simulink model "CH"  (R2024a)
settings: Solver=VariableStepAuto  StartTime=0.0  StopTime=7000  FixedStep=1e-3  RelTol=1e-3
libraries: visionfilter x1, commrandsrc3 x1
(part 1 of 3)
settings Model: Creator=Eng. Amr  LastModifiedBy=Eng. Amr

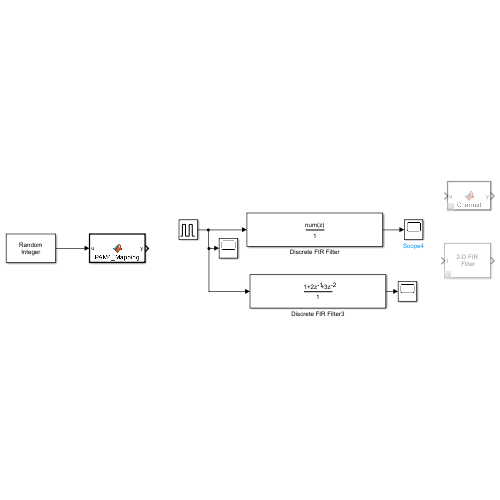
[thumbnail: Simulink's stored preview of the top-level diagram]
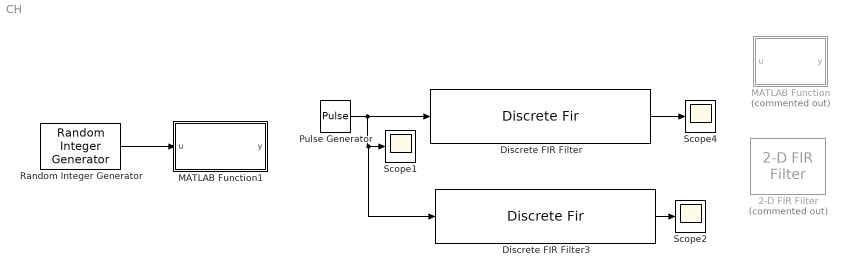
== system CH ==
  2-D FIR Filter : visionfilter/2-D FIR Filter  Commented=on  separable=off  filtSrc=Specify via dialog  filterMtrx=[1 0; 0 -1]  verticalFilter=[4 0]  horizontalFilter=[4 0]  outSize=Full  padType=Constant  padSrc=Specify via dialog  padVal=0  method=Convolution  firstCoeffMode=Specify word length  firstCoeffWordLength=16  firstCoeffFracLength=14  firstCoeffSignedness=Signed  firstCoeffLastDataTypeStr=fixdt(1,16)  outputSignedness=Auto  accumLastDataTypeStr=Inherit: Same as product output  prodOutputMode=Binary point scaling  prodOutputWordLength=32  prodOutputFracLength=10  prodOutputLastDataTypeStr=fixdt([],32,10)  roundingMode=Floor  overflowMode=off  firstCoeffDataTypeStr=fixdt(1,16)  firstCoeffMin=[]  firstCoeffMax=[]  prodOutputDataTypeStr=fixdt([],32,10)  accumDataTypeStr=Inherit: Same as product output  outputMin=[]  outputMax=[]
  Discrete FIR Filter : DiscreteFir  Coefficients=[0.000082081 0.000081826 0.000082747 0.000085619 0.000087998 0.000088639 0.000089241 0.000089656 0.000088480 0.000087334 0.000087328 0.000086157 0.000084826 0.000085166 0.000086761 0.000088856 0.000091646 0.000094652 0.000095475 0.000091876 0.000085087 0.000077981 0.000071874 0.000069173 0.000071497 0.000076858 0.000081323 0.000085713 0.000087545 0.000083688 0.000076042 0.000066245 0.000055538 0.000047208 0.000044183 0.000048550 0.000062019 0.000080085 0.000095608 0.000104279 0.000105476 0.000098162 0.000085768 0.000076525 0.000073439 0.000079441 0.000094448 0.000117739 0.000145078 0.000166000 0.000175965 0.000170331 0.000147135 0.000110978 0.000075440 0.000047221 0.000030509 0.000027282 0.000037581 0.000042702 0.000039947 0.000038432 0.000033646 0.000020941 0.000010243 0.000007172 0.000013032 0.000022489 0.000035128 0.000067418 0.000117313 0.000148686 0.000179558 0.000226378 0.000266266 0.000286140 0.000281862 0.000245316 0.000172933 0.000075379 -0.000032035 -0.000122022 -0.000172531 -0.000172558 -0.000123911 -0.000050997 0.000015362 0.000074030 0.000126520 0.000169663 0.000197846 0.000233481 0.000275516 0.000281279 0.000228408 0.000138428 0.000042774 -0.000017693 -0.000052514 -0.000052926 -0.000006045 0.000058139 0.000076225 0.000065879 0.000065356 0.000076336 0.000099974 0.000125440 0.000142716 0.000147540 0.000133622 0.000102034 0.000066605 0.000040570 0.000042604 0.000063494 0.000086879 0.000093660 0.000090577 0.000086015 0.000076983 0.000067972 0.000072415 0.000093143 0.000108892 0.000102521 0.000081429 0.000066589 0.000075000 0.000085753 0.000086147 0.000084813 0.000084217 0.000083891 0.000083706 0.000083680 0.000083751 0.000083820 0.000083832 0.000083800 0.000083769 0.000083770 0.000083795 0.000083817 0.000083819 0.000083805 0.000083794 0.000083795 0.000083806 0.000083815 0.000083814 0.000083806 0.000083803 0.000083810 0.000083822 0.000083831 0.000083831 0.000083826 0.000083824 0.000083828 0.000083834 0.000083837 0.000083833 0.000083828 0.000083828 0.000083834 0.000083842 0.000083847 0.000083847 0.000083844 0.000083843 0.000083845 0.000083845 0.000083845 0.000083841 0.000083837 0.000083837 0.000083841 0.000083845 0.000083847 0.000083846 0.000083844 0.000083844 0.000083844 0.000083843 0.000083842 0.000083838 0.000083834 0.000083833 0.000083835 0.000083839 0.000083842 0.000083843 0.000083842 0.000083842 0.000083843 0.000083844 0.000083843 0.000083840 0.000083837 0.000083839 0.000083843 0.000083847 0.000083850 0.000083852 0.000083854 0.000083858 0.000083860 0.000083862 0.000083862 0.000083861 0.000083860 0.000083862 0.000083865 0.000083868 0.000083873 0.000083878 0.000083881 0.000083883 0.000083885 0.000083887 0.000083889 0.000083888 0.000083885 0.000083885 0.000083888 0.000083891 0.000083895 0.000083897 0.000083898 0.000083901 0.000083904 0.000083905 0.000083903 0.000083897 0.000083894 0.000083894 0.000083895 0.000083896 0.000083897 0.000083897 0.000083898 0.000083900 0.000083902 0.000083901 0.000083898 0.000083894 0.000083891 0.000083890 0.000083890 0.000083890 0.000083893 0.000083896 0.000083899 0.000083903 0.000083905 0.000083905 0.000083905 0.000083903 0.000083902 0.000083903 0.000083903 0.000083905 0.000083908 0.000083911 0.000083914 0.000083919 0.000083922 0.000083924 0.000083923 0.000083920 0.000083917 0.000083918 0.000083920 0.000083922 0.000083926 0.000083930 0.000083935 0.000083944 0.000083951 0.000083954 0.000083957 0.000083957 0.000083957 0.000083958 0.000083958 0.000083959 0.000083962 0.000083965 0.000083968 0.000083972 0.000083973 0.000083971 0.000083967 0.000083959 0.000083951 0.000083945 0.000083940 0.000083937 0.000083938 0.000083940 0.000083946 0.000083957 0.000083969 0.000083977 0.000083984 0.000083986 0.000083986 0.000083987 0.000083984 0.000083978 0.000083972 0.000083966 0.000083965 0.000083967 0.000083967 0.000083964 0.000083960 0.000083954 0.000083948 0.000083942 0.000083936 0.000083933 0.000083937 0.000083946 0.000083962 0.000083984 0.000084005 0.000084027 0.000084049 0.000084064 0.000084070 ...(+28772 chars)]
  Discrete FIR Filter3 : DiscreteFir  Coefficients=[1 2 3]
  MATLAB Function : MATLAB Function  Commented=on  TreatAsAtomicUnit=on
  MATLAB Function1 : MATLAB Function  TreatAsAtomicUnit=on
  Pulse Generator : DiscretePulseGenerator  PulseType=Time based  Period=7000  PulseWidth=20
  Random Integer Generator : commrandsrc3/Random Integer Generator  SetSize=4  SeedSource=Auto  Seed=0  SampleTime=1  SamplesPerFrame=1  OutputDataType=uint8  SimulateUsing=Interpreted execution
  Scope1 : Scope
  Scope2 : Scope
  Scope4 : Scope
  wires:
  Random Integer Generator/1 -> MATLAB Function1/1(u)
  Discrete FIR Filter/1 -> Scope4/1
  Pulse Generator/1 -> Discrete FIR Filter3/1, Scope1/1, Discrete FIR Filter/1
  Discrete FIR Filter3/1 -> Scope2/1
